simulink model "suficiencia_CD"  (R2024a)
settings: Solver=FixedStepAuto  StartTime=0.0  StopTime=400  FixedStep=Ts/20  RelTol=1e-3
undefined symbols (not defined in the file): K, q0_pi, q0_pi_cr, q0_pi_s, q0_pid, q0_pid_cr, q1_pi, q1_pi_cr, q1_pi_s, q1_pid, q1_pid_cr, q2, q2_cr, tau, Ts
libraries: simulink x3

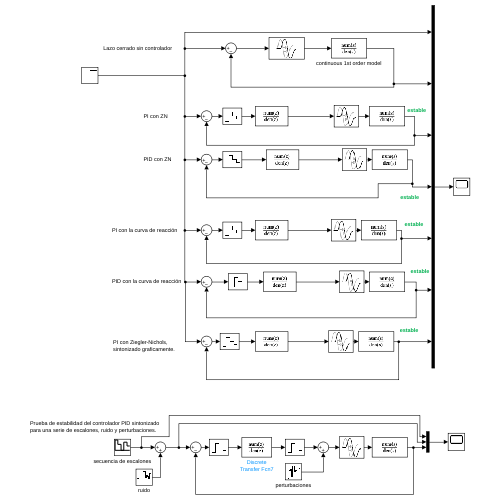
[thumbnail: Simulink's stored preview of the top-level diagram]
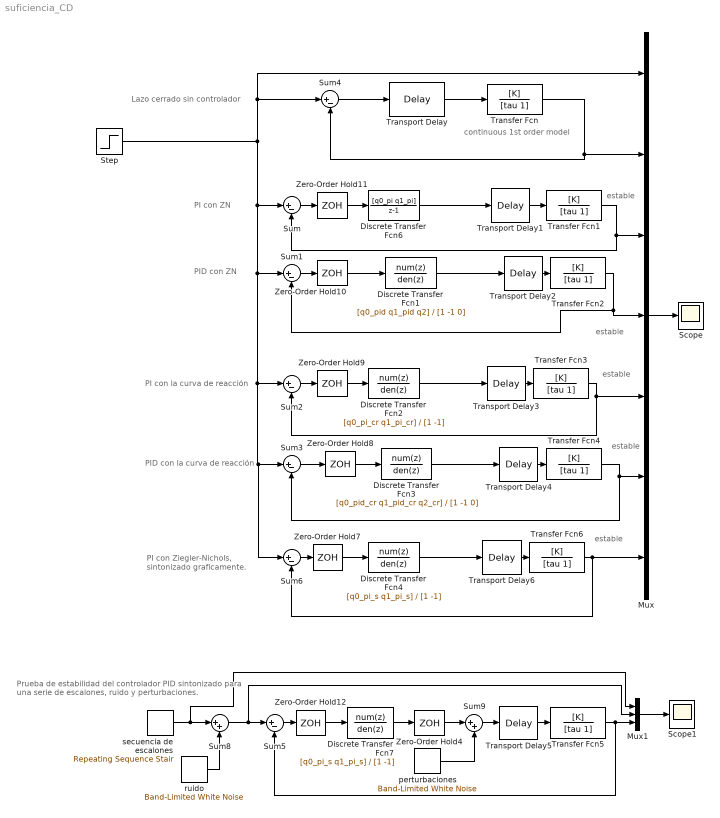
== system suficiencia_CD ==
  note: estable
  note: Lazo cerrado sin controlador
  note: PI con ZN
  note: continuous 1st order model
  note: PID con ZN
  note: PID con la curva de reacción
  note: PI con la curva de reacción
  note: estable
  note: estable
  note: PI con Ziegler-Nichols,
      | sintonizado graficamente.
  note: Prueba de estabilidad del controlador PID sintonizado
      | para una serie de escalones, ruido y perturbaciones.
  note: estable
  note: estable
  Discrete Transfer Fcn1 : DiscreteTransferFcn  Numerator=[q0_pid q1_pid q2]  Denominator=[1 -1 0]
  Discrete Transfer Fcn2 : DiscreteTransferFcn  Numerator=[q0_pi_cr q1_pi_cr]  Denominator=[1 -1]
  Discrete Transfer Fcn3 : DiscreteTransferFcn  Numerator=[q0_pid_cr q1_pid_cr q2_cr]  Denominator=[1 -1 0]
  Discrete Transfer Fcn4 : DiscreteTransferFcn  Numerator=[q0_pi_s q1_pi_s]  Denominator=[1 -1]
  Discrete Transfer Fcn6 : DiscreteTransferFcn  Numerator=[q0_pi q1_pi]  Denominator=[1 -1]
  Discrete Transfer Fcn7 : DiscreteTransferFcn  Numerator=[q0_pi_s q1_pi_s]  Denominator=[1 -1]
  Mux : Mux  Inputs=7
  Mux1 : Mux  Inputs=3
  Scope : Scope
  Scope1 : Scope
  Step : Step  SampleTime=0
  Sum{,1..6} (7 alike) : Sum  Inputs=|+-
  Sum8 : Sum  Inputs=|++
  Sum9 : Sum  Inputs=|++
  Transfer Fcn{,1..6} (7 alike) : TransferFcn  Numerator=[K]  Denominator=[tau 1]
  Transport Delay{,1..6} (7 alike) : TransportDelay  DelayTime=2.2
  Zero-Order Hold{4,7..12} (7 alike) : ZeroOrderHold  SampleTime=Ts
  perturbaciones : simulink/Sources/Band-Limited White Noise  Cov=[0.3]  Ts=10*Ts  seed=[23341]
  ruido : simulink/Sources/Band-Limited White Noise  Cov=[0.1]  Ts=Ts/10  seed=[23341]
  secuencia de escalones : simulink/Sources/Repeating Sequence Stair  OutValues=[5 3 0 4 2].'  tsamp=10*Ts  OutMin=[]  OutMax=[]  OutDataTypeStr=double  OutputDataTypeScalingMode=double  OutDataType=fixdt(0,8)  ConRadixGroup=Best Precision: Vector-wise  OutScaling=2^-12
  wires:
  Transport Delay/1 -> Transfer Fcn/1
  Transfer Fcn/1 -> Sum4/2, Mux/2
  Transfer Fcn2/1 -> Mux/4, Sum1/2
  Transport Delay1/1 -> Transfer Fcn1/1
  Discrete Transfer Fcn6/1 -> Transport Delay1/1
  Sum/1 -> Zero-Order Hold11/1
  Sum1/1 -> Zero-Order Hold10/1
  Transport Delay2/1 -> Transfer Fcn2/1
  Transfer Fcn3/1 -> Mux/5, Sum2/2
  Discrete Transfer Fcn2/1 -> Transport Delay3/1
  Sum2/1 -> Zero-Order Hold9/1
  Transport Delay3/1 -> Transfer Fcn3/1
  Transport Delay4/1 -> Transfer Fcn4/1
  Transfer Fcn4/1 -> Mux/6, Sum3/2
  Discrete Transfer Fcn3/1 -> Transport Delay4/1
  Sum3/1 -> Zero-Order Hold8/1
  Transfer Fcn1/1 -> Mux/3, Sum/2
  Sum4/1 -> Transport Delay/1
  Transport Delay6/1 -> Transfer Fcn6/1
  Transfer Fcn6/1 -> Mux/7, Sum6/2
  Step/1 -> Mux/1, Sum4/1, Sum6/1, Sum3/1, Sum2/1, Sum1/1, Sum/1
  Mux/1 -> Scope/1
  Transport Delay5/1 -> Transfer Fcn5/1
  Discrete Transfer Fcn7/1 -> Zero-Order Hold4/1
  Transfer Fcn5/1 -> Mux1/3, Sum5/2
  Mux1/1 -> Scope1/1
  Sum6/1 -> Zero-Order Hold7/1
  Zero-Order Hold7/1 -> Discrete Transfer Fcn4/1
  Zero-Order Hold8/1 -> Discrete Transfer Fcn3/1
  Zero-Order Hold9/1 -> Discrete Transfer Fcn2/1
  Zero-Order Hold10/1 -> Discrete Transfer Fcn1/1
  Zero-Order Hold11/1 -> Discrete Transfer Fcn6/1
  Sum5/1 -> Zero-Order Hold12/1
  Zero-Order Hold12/1 -> Discrete Transfer Fcn7/1
  secuencia de escalones/1 -> Mux1/1, Sum8/1
  Sum8/1 -> Mux1/2, Sum5/1
  ruido/1 -> Sum8/2
  Zero-Order Hold4/1 -> Sum9/1
  Sum9/1 -> Transport Delay5/1
  perturbaciones/1 -> Sum9/2
  Discrete Transfer Fcn1/1 -> Transport Delay2/1
  Discrete Transfer Fcn4/1 -> Transport Delay6/1
